simulink model "Square_HFI"  (R2022b)
settings: Solver=FixedStepAuto  StartTime=0.0  StopTime=10  FixedStep=1e-5  RelTol=1e-3
undefined symbols (not defined in the file): curr_d_ki, curr_d_kp, curr_q_ki, curr_q_kp, CurrKi, CurrKpd, CurrKpq, DiscIntNeverNeededParam, Ld, Lq, PLL_Kd, PLL_Ki, Pn, sigbuilder_block, spd_ki, spd_kp
libraries: dsparch4 x4, slpidlib x3, mcbplantlib x1, autolibpmsminterior x1, autolibpmsmexterior x1
settings Model: DataDictionary=Square_HFI.sldd  Creator=SSC  LastModifiedBy=SSC
settings GRTTargetCC: RTWCAPISignals=on  RTWCAPIParams=on

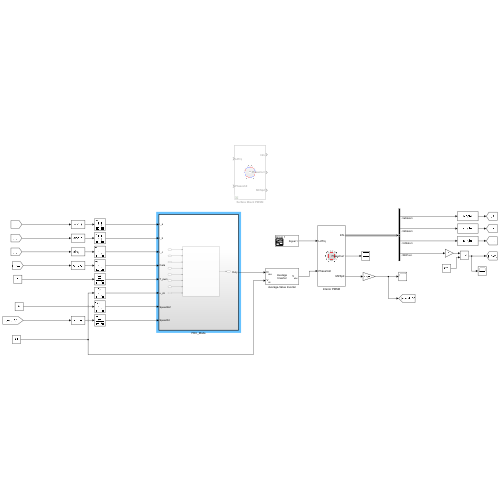
[thumbnail: Simulink's stored preview of the top-level diagram]
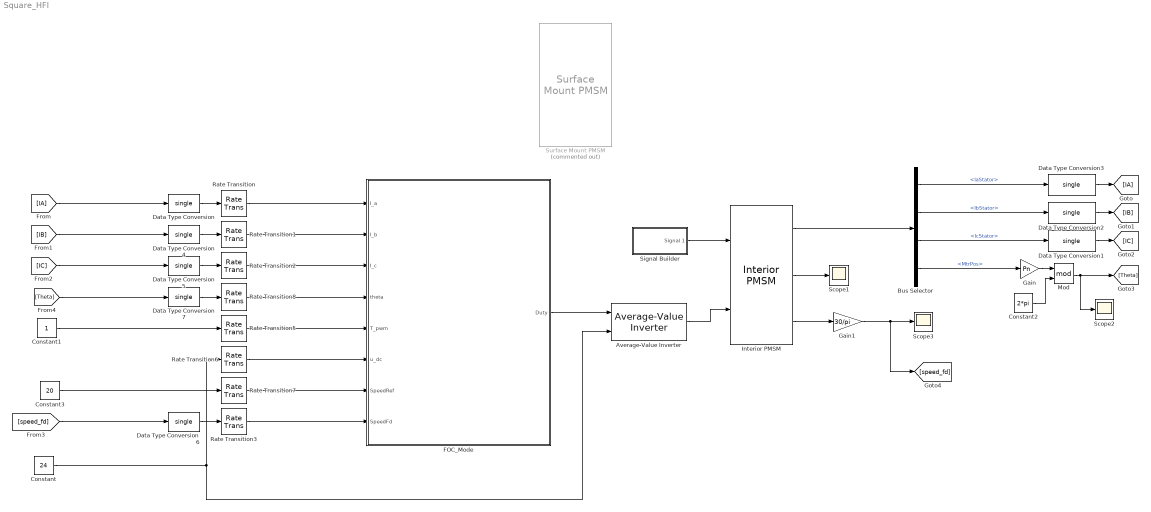
== system Square_HFI ==
  Average-Value Inverter : mcbplantlib/Average-Value Inverter
      settings: LibrarySourceBlock=mcblib/Electrical Systems/Inverters/Average-Value Inverter
  Bus Selector : BusSelector  OutputSignals=IaStator,IbStator,IcStator,MtrPos
  Constant : Constant  Value=24  OutDataTypeStr=single
  Constant1 : Constant  OutDataTypeStr=single
  Constant2 : Constant  Value=2*pi  OutDataTypeStr=single
  Constant3 : Constant  Value=20  OutDataTypeStr=single
  Data Type Conversion{,1..7} (8 alike) : DataTypeConversion  OutDataTypeStr=single  SaturateOnIntegerOverflow=off  RndMeth=Floor
  FOC_Mode : Subsystem  TreatAsAtomicUnit=on
  Gain : Gain  Gain=Pn  OutDataTypeStr=single
  Gain1 : Gain  Gain=30/pi  OutDataTypeStr=single
  Interior PMSM : autolibpmsminterior/Interior PMSM  port_config=Torque  sim_type=Discrete  Ts=1e-4  P=Pn  Rs=Rs  Ldq=[Ld Lq]  KConstText=Permanent flux linkage constant (lambda_pm):  lambda_pm=flux  Ke=159.9771  mechanical=[75e-6,8e-5,0]  idq0=[0 0]  theta_init=0  omega_init=0  KConst=flux  lambda_pm_calc=flux  Kt=0.07  RefBlkName='autolibpmsminterior/Interior PMSM'  aMode=5
      settings: LibrarySourceBlock=mcblib/Electrical Systems/Motors/Interior PMSM
  Mod : Math  Operator=mod
  Rate Transition{,1..3,5..8} (8 alike) : RateTransition
  Scope1 : Scope
  Scope2 : Scope
  Scope3 : Scope
  Signal Builder : Subsystem  Tag=STV Subsys  LoadFcn=sigbuilder_block('load');  StartFcn=sigbuilder_block('start');  StopFcn=sigbuilder_block('stop');  ClipboardFcn=sigbuilder_block('clipboard');  mask(Sigbuilder block){tuvar=[0:10]}
      mask help: Simulink:masks:SigbuilderBlock_MD
      mask init:
      | if ~strcmp(get_param(bdroot(gcbh),'SimulationStatus'),'stopped') tuvar = sigbuilder_block('maskInit'); end
      settings: CopyFcn=sigbuilder_block('copy');  DeleteFcn=sigbuilder_block('delete');  ModelCloseFcn=sigbuilder_block('modelClose');  PreSaveFcn=sigbuilder_block('preSave');  PauseFcn=sigbuilder_block('pause');  ContinueFcn=sigbuilder_block('continue');  NameChangeFcn=sigbuilder_block('namechange');  OpenFcn=sigbuilder_block('open',[367.2 103.2 550.8 400.2 ]);  CloseFcn=sigbuilder_block('close');
      mask Display: plot(0, 0, 100, 100,[2, 2, 32, 32, 2], [68, 8, 8, 68, 68],[32, 2], [38, 38], [32, 19, 2],[53, 60, 44], [32, 17, 17, 2],[16, 16, 31, 31]);txt = getActiveGroup(gcbh);text(2, 100, txt,'verticalAlignment', 'top');
  Surface Mount PMSM : autolibpmsmexterior/Surface Mount PMSM  Commented=on  port_config=Torque  sim_type=Discrete  Ts=1e-4  P=Pn  Rs=Rs  Ldq_=Ld  KConstText=Permanent flux linkage constant (lambda_pm):  lambda_pm=flux  Ke=223  Kt=1.323  mechanical=[75e-6,8e-5,0]  idq0=[0 0]  theta_init=0  omega_init=0  KConst=flux  lambda_pm_calc=flux  RefBlkName='autolibpmsmexterior/Surface Mount PMSM'  aMode=5  Ldq="[0.0017      0.0017]"
  wires:
  Rate Transition/1 -> FOC_Mode/1(I_a)
  Average-Value Inverter/1 -> Interior PMSM/2
  Rate Transition7/1 -> FOC_Mode/7(SpeedRef)
  Data Type Conversion6/1 -> Rate Transition3/1
  [IC] -> Data Type Conversion5/1
  Data Type Conversion5/1 -> Rate Transition2/1
  Data Type Conversion2/1 -> [IB]
  Rate Transition1/1 -> FOC_Mode/2(I_b)
  Interior PMSM/2 -> Scope1/1
  Bus Selector/3 -> Data Type Conversion1/1  "<IcStator>"
  Rate Transition6/1 -> FOC_Mode/6(u_dc)
  Constant1/1 -> Rate Transition5/1
  Bus Selector/4 -> Gain/1  "<MtrPos>"
  FOC_Mode/1(Duty) -> Average-Value Inverter/1
  [IA] -> Data Type Conversion/1
  Gain1/1 -> Scope3/1, [speed_fd]
  Rate Transition8/1 -> FOC_Mode/4(theta)
  Bus Selector/2 -> Data Type Conversion2/1  "<IbStator>"
  Data Type Conversion/1 -> Rate Transition/1
  Interior PMSM/1 -> Bus Selector/1
  Data Type Conversion3/1 -> [IA]
  Interior PMSM/3 -> Gain1/1
  Constant3/1 -> Rate Transition7/1
  Gain/1 -> Mod/1
  [Theta] -> Data Type Conversion7/1
  Rate Transition2/1 -> FOC_Mode/3(I_c)
  Data Type Conversion4/1 -> Rate Transition1/1
  Bus Selector/1 -> Data Type Conversion3/1  "<IaStator>"
  [speed_fd] -> Data Type Conversion6/1
  Data Type Conversion7/1 -> Rate Transition8/1
  Mod/1 -> Scope2/1, [Theta]
  Rate Transition3/1 -> FOC_Mode/8(SpeedFd)
  Constant/1 -> Average-Value Inverter/2, Rate Transition6/1
  Constant2/1 -> Mod/2
  Data Type Conversion1/1 -> [IC]
  Rate Transition5/1 -> FOC_Mode/5(T_pwm)
  [IB] -> Data Type Conversion4/1
  Signal Builder/1(Signal 1) -> Interior PMSM/1

== system Square_HFI/FOC_Mode ==
  I_a : Inport
  I_b : Inport  Port=2
  I_c : Inport  Port=3
  theta : Inport  Port=4
  T_pwm : Inport  Port=5
  u_dc : Inport  Port=6
  SpeedRef : Inport  Port=7
  SpeedFd : Inport  Port=8
  HFI_Mode : Subsystem  TreatAsAtomicUnit=on
  Duty : Outport
  wires:
  T_pwm/1 -> HFI_Mode/5(T_pwm)
  u_dc/1 -> HFI_Mode/6(u_dc)
  HFI_Mode/1(Duty) -> Duty/1
  I_a/1 -> HFI_Mode/1(I_a)
  I_b/1 -> HFI_Mode/2(I_b)
  I_c/1 -> HFI_Mode/3(I_c)
  theta/1 -> HFI_Mode/4(theta)
  SpeedRef/1 -> HFI_Mode/7(SpeedRef)
  SpeedFd/1 -> HFI_Mode/8(SpeedFd)

== system Square_HFI/Signal Builder ==
  Demux : Demux  Tag=STV Demux  Outputs=1
      settings: DisplayOption=none
  FromWs : FromWorkspace  Tag=STV FromWs  VariableName=tuvar
      SigBuilderData=|
      | common.afterFinalStr = 'Extrapolate'
      | common.sampleTime = 0
      | dataSet.timeRange = [0 10]
      | dataSet.name = 'Group 1'
      | sbobj.Groups.Name = 'Group 1'
      | sbobj.Groups.Signals.Name = 'Signal 1'
      | sbobj.Groups.Signals.XData = [0 4 4 6 10]
      | sbobj.Groups.Signals.YData = [0 0 0.0003 0.0003 0.0003]
  Signal 1 : Outport  Tag=STV Outport
  wires:
  Demux/1 -> Signal 1/1
  FromWs/1 -> Demux/1

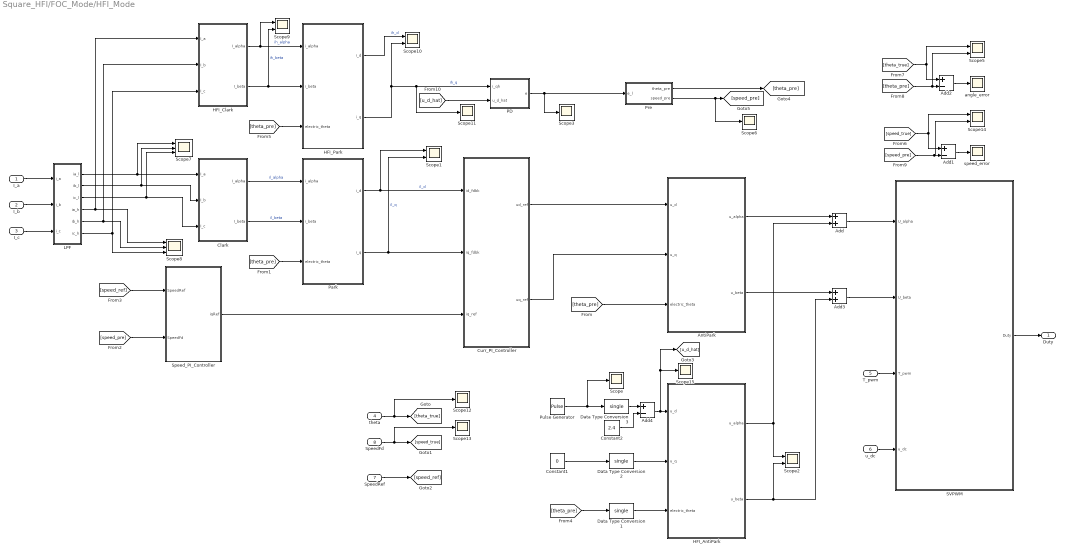
== system Square_HFI/FOC_Mode/HFI_Mode ==
  I_a : Inport
  I_b : Inport  Port=2
  I_c : Inport  Port=3
  theta : Inport  Port=4
  T_pwm : Inport  Port=5
  u_dc : Inport  Port=6
  SpeedRef : Inport  Port=7
  SpeedFd : Inport  Port=8
  Add : Sum  OutDataTypeStr=single
  Add1 : Sum  Inputs=+-  OutDataTypeStr=single
  Add2 : Sum  Inputs=+-  OutDataTypeStr=single
  Add3 : Sum  OutDataTypeStr=single
  Add4 : Sum  Inputs=+-  OutDataTypeStr=single
  AntiPark : Subsystem
  Clark : Subsystem
  Constant1 : Constant  Value=0  OutDataTypeStr=single
  Constant2 : Constant  Value=2.4  OutDataTypeStr=single
  Curr_PI_Controller : Subsystem
  Data Type Conversion1 : DataTypeConversion  OutDataTypeStr=single  SaturateOnIntegerOverflow=off  RndMeth=Floor
  Data Type Conversion2 : DataTypeConversion  OutDataTypeStr=single  SaturateOnIntegerOverflow=off  RndMeth=Floor
  Data Type Conversion3 : DataTypeConversion  OutDataTypeStr=single  SaturateOnIntegerOverflow=off  RndMeth=Floor
  HFI_AntiPark : Subsystem
  HFI_Clark : Subsystem
  HFI_Park : Subsystem
  LPF : Subsystem
  PD : Subsystem
  Park : Subsystem
  Pre : Subsystem
  Pulse Generator : DiscretePulseGenerator  PulseType=Time based  Amplitude=4.8  Period=0.001  PulseWidth=50
  SVPWM : Subsystem
  Scope{,3,6,11..13,15} (7 alike) : Scope
  Scope{1..2,5,9..10,14} (6 alike) : Scope  NumInputPorts=2
  Scope7 : Scope  NumInputPorts=3
  Scope8 : Scope  NumInputPorts=3
  Speed_PI_Controller : Subsystem
  angle_error : Scope
  speed_error : Scope
  Duty : Outport
  wires:
  Curr_PI_Controller/2(uq_ref) -> AntiPark/2(u_q)
  SVPWM/1(Duty) -> Duty/1
  u_dc/1 -> SVPWM/4(u_dc)
  T_pwm/1 -> SVPWM/3(T_pwm)
  Curr_PI_Controller/1(ud_ref) -> AntiPark/1(u_d)
  PD/1(e) -> Pre/1(e_l), Scope3/1
  Pulse Generator/1 -> Scope/1, Data Type Conversion3/1
  Add/1 -> SVPWM/1(U_alpha)
  Add3/1 -> SVPWM/2(U_beta)
  Constant1/1 -> Data Type Conversion2/1
  I_b/1 -> LPF/2(i_b)
  I_a/1 -> LPF/1(i_a)
  I_c/1 -> LPF/3(i_c)
  AntiPark/1(u_alpha) -> Add/1
  AntiPark/2(u_beta) -> Add3/1
  theta/1 -> Scope12/1, [theta_true]
  SpeedFd/1 -> Scope13/1, [speed_true]
  Park/1(i_d) -> Scope1/1, Curr_PI_Controller/1(id_fdbk)  "il_d"
  Park/2(i_q) -> Scope1/2, Curr_PI_Controller/2(iq_fdbk)  "il_q"
  Speed_PI_Controller/1(iqRef) -> Curr_PI_Controller/3(iq_ref)
  [theta_pre] -> AntiPark/3(electric_theta)
  Clark/1(I_alpha) -> Park/1(i_alpha)  "il_alpha"
  Clark/2(I_beta) -> Park/2(i_beta)  "il_beta"
  [theta_pre] -> Park/3(electric_theta)
  LPF/1(ia_l) -> Scope7/1, Clark/1(I_a)
  LPF/3(ic_l) -> Scope7/3, Clark/3(I_c)
  LPF/2(ib_l) -> Scope7/2, Clark/2(I_b)
  [speed_pre] -> Speed_PI_Controller/2(SpeedFd)
  SpeedRef/1 -> [speed_ref]
  [speed_ref] -> Speed_PI_Controller/1(SpeedRef)
  [theta_pre] -> Data Type Conversion1/1
  HFI_AntiPark/1(u_alpha) -> Add/2, Scope2/1
  HFI_AntiPark/2(u_beta) -> Add3/2, Scope2/2
  LPF/4(ia_h) -> HFI_Clark/1(I_a), Scope8/1
  LPF/5(ib_h) -> HFI_Clark/2(I_b), Scope8/2
  LPF/6(ic_h) -> Scope8/3, HFI_Clark/3(I_c)
  HFI_Clark/1(I_alpha) -> HFI_Park/1(i_alpha), Scope9/1  "ih_alpha"
  HFI_Clark/2(I_beta) -> HFI_Park/2(i_beta), Scope9/2  "ih_beta"
  [theta_pre] -> HFI_Park/3(electric_theta)
  HFI_Park/1(i_d) -> Scope10/1  "ih_d"
  HFI_Park/2(i_q) -> Scope10/2, Scope11/1, PD/1(i_qh)  "ih_q"
  Pre/2(speed_pre) -> Scope6/1, [speed_pre]
  Pre/1(theta_pre) -> [theta_pre]
  [theta_pre] -> Scope5/2, Add2/2
  [theta_true] -> Add2/1, Scope5/1
  Add2/1 -> angle_error/1
  Data Type Conversion1/1 -> HFI_AntiPark/3(electric_theta)
  Data Type Conversion2/1 -> HFI_AntiPark/2(u_q)
  [speed_true] -> Scope14/1, Add1/1
  [speed_pre] -> Scope14/2, Add1/2
  Add1/1 -> speed_error/1
  Data Type Conversion3/1 -> Add4/1
  Add4/1 -> [u_d_hat], Scope15/1, HFI_AntiPark/1(u_d)
  Constant2/1 -> Add4/2
  [u_d_hat] -> PD/2(u_d_hat)

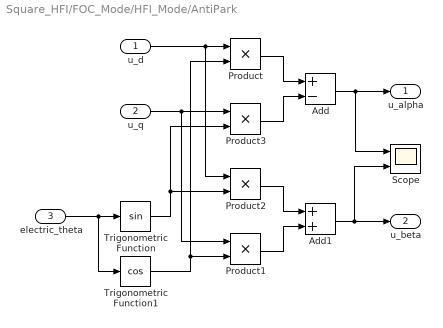
== system Square_HFI/FOC_Mode/HFI_Mode/AntiPark ==
  u_d : Inport
  u_q : Inport  Port=2
  electric_theta : Inport  Port=3
  Add : Sum  Inputs=+-
  Add1 : Sum
  Product{,1..3} (4 alike) : Product
  Scope : Scope  NumInputPorts=2
  Trigonometric Function : Trigonometry
  Trigonometric Function1 : Trigonometry  Operator=cos
  u_alpha : Outport
  u_beta : Outport  Port=2
  wires:
  electric_theta/1 -> Trigonometric Function1/1, Trigonometric Function/1
  u_d/1 -> Product2/1, Product/1
  Trigonometric Function1/1 -> Product/2, Product1/2
  u_q/1 -> Product1/1, Product3/1
  Trigonometric Function/1 -> Product2/2, Product3/2
  Product/1 -> Add/1
  Product3/1 -> Add/2
  Add/1 -> Scope/1, u_alpha/1
  Product2/1 -> Add1/1
  Product1/1 -> Add1/2
  Add1/1 -> Scope/2, u_beta/1

== system Square_HFI/FOC_Mode/HFI_Mode/Clark ==
  I_a : Inport
  I_b : Inport  Port=2
  I_c : Inport  Port=3
  Add : Sum
  Add1 : Sum  Inputs=+-
  Add2 : Sum  Inputs=+-
  Gain : Gain  Gain=2/3
  Gain1 : Gain  Gain=1/3
  Gain2 : Gain  Gain=sqrt(3)/3
  I_alpha : Outport
  I_beta : Outport  Port=2
  wires:
  I_a/1 -> Gain/1
  I_b/1 -> Add1/1, Add/1
  I_c/1 -> Add/2, Add1/2
  Add/1 -> Gain1/1
  Add1/1 -> Gain2/1
  Gain/1 -> Add2/1
  Gain1/1 -> Add2/2
  Add2/1 -> I_alpha/1
  Gain2/1 -> I_beta/1

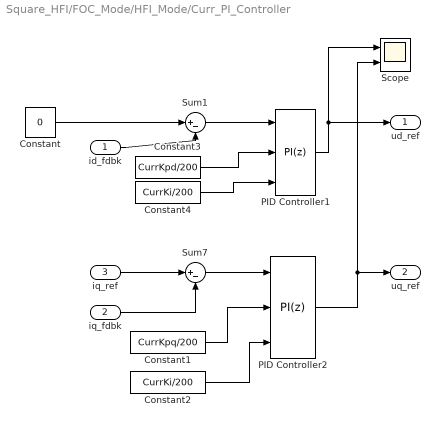
== system Square_HFI/FOC_Mode/HFI_Mode/Curr_PI_Controller ==
  id_fdbk : Inport  OutDataTypeStr=single
  iq_fdbk : Inport  Port=2  OutDataTypeStr=single
  iq_ref : Inport  Port=3  OutDataTypeStr=single
  Constant : Constant  Value=0  OutDataTypeStr=single
  Constant1 : Constant  Value=CurrKpq/200  OutDataTypeStr=single
  Constant2 : Constant  Value=CurrKi/200  OutDataTypeStr=single
  Constant3 : Constant  Value=CurrKpd/200  OutDataTypeStr=single
  Constant4 : Constant  Value=CurrKi/200  OutDataTypeStr=single
  PID Controller1 : slpidlib/PID Controller  Controller=PI  Form=Parallel  TimeDomain=Discrete-time  UseExternalTs=off  SampleTime=-1  IntegratorMethod=Forward Euler  FilterMethod=Forward Euler  ControllerParametersSource=external  P=curr_d_kp  I=curr_d_ki  UseKiTs=off  D=0  N=100  UseFilter=on  TunerSelectOption=Transfer Function Based (PID Tuner App)  InitialConditionSource=internal  InitialConditionForIntegrator=0  InitialConditionForFilter=0  DifferentiatorICPrevScaledInput=0  ExternalReset=none  TrackingMode=off  Kt=1  LimitOutput=on  SatLimitsSource=internal  UpperSaturationLimit=24*0.9/sqrt(3)  LowerSaturationLimit=-24*0.9/sqrt(3)  LinearizeAsGain=on  AntiWindupMode=clamping  Kb=1  LimitIntegrator=off  UpperIntegratorSaturationLimit=inf  LowerIntegratorSaturationLimit=-inf  PGainOutDataTypeStr=single  PProdOutDataTypeStr=single  POutMin=[]  POutMax=[]  IGainOutDataTypeStr=int16  IProdOutDataTypeStr=int16  IOutMin=[]  IOutMax=[]  DOutMin=[]  DOutMax=[]  NOutMin=[]  NOutMax=[]  SumOutDataTypeStr=single  SumOutMin=[]  SumOutMax=[]  SaturationOutDataTypeStr=single  SaturationOutMin=[]  SaturationOutMax=[]  PParamMin=[]  PParamMax=[]  IParamMin=[]  IParamMax=[]  DParamMin=[]  DParamMax=[]  NParamMin=[]  NParamMax=[]  KbParamMin=[]  KbParamMax=[]  KtParamMin=[]  KtParamMax=[]  KbOutMin=[]  KbOutMax=[]  KtOutMin=[]  KtOutMax=[]  IntegratorOutMin=[]  IntegratorOutMax=[]  FilterOutMin=[]  FilterOutMax=[]  SumI1OutMin=[]  SumI1OutMax=[]  SumI2OutMin=[]  SumI2OutMax=[]  SumI3OutMin=[]  SumI3OutMax=[]  SumI4OutMin=[]  SumI4OutMax=[]  SumDOutMin=[]  SumDOutMax=[]  DifferentiatorOutMin=[]  DifferentiatorOutMax=[]  FilterDiffOutCoefMin=[]  FilterDiffOutCoefMax=[]  ReciprocalOutMin=[]  ReciprocalOutMax=[]  SumDenOutMin=[]  SumDenOutMax=[]  SumNumOutMin=[]  SumNumOutMax=[]  DivideOutMin=[]  DivideOutMax=[]  UdiffTsProdOutMin=[]  UdiffTsProdOutMax=[]  NTsProdOutMin=[]  NTsProdOutMax=[]  UintegralTsProdOutMin=[]  UintegralTsProdOutMax=[]  UngainTsProdOutMin=[]  UngainTsProdOutMax=[]  ClampingZeroOutDataTypeStr=Inherit: Inherit via back propagation  ClampingZeroOutMin=[]  ClampingZeroOutMax=[]  FilterDenConstantOutDataTypeStr=Inherit: Inherit via back propagation  FilterDenConstantOutMin=[]  FilterDenConstantOutMax=[]  PCopyOutDataTypeStr=Inherit: Inherit via back propagation  PCopyOutMin=[]  PCopyOutMax=[]  NCopyOutDataTypeStr=Inherit: Inherit via back propagation  NCopyOutMin=[]  NCopyOutMax=[]  IntegratorContinuousStateAttributes=''  IntegratorStateMustResolveToSignalObject=off  IntegratorRTWStateStorageClass=Auto  FilterContinuousStateAttributes=''  FilterStateMustResolveToSignalObject=off  FilterRTWStateStorageClass=Auto  ParallelPVariant=ExternalParameters  IdealPVariant=Disabled  IVariant=ExternalParameters  DVariant=Disabled  IntegratorVariant=Discrete  SatVariant=Enabled  AWVariant=DiscClampingParallel  PCopyVariant=Disabled  TRVariant=Disabled  FdbkBlocksVariant=Forward  IdealPFdbkVariant=Disabled  SatFdbkVariant=Disabled  DerivativeFilterVariant=Disabled  NVariant=Disabled  NCopyVariant=Disabled_SignalSpec  FilterICVariant=Disabled  IntegratorICVariant=InternalICs  ExternalResetVariant=Disabled  TRSumVariant=Passthrough  SumFdbkVariant=Disabled  SumVariant=Sum_PI  TsampFilterVariant=InternalTs  TsampNgainVariant=Passthrough  TsampIntegralVariant=Passthrough  ExternalSaturationOutDataTypeStr=Inherit: Same as second input
  PID Controller2 : slpidlib/PID Controller  Controller=PI  Form=Parallel  TimeDomain=Discrete-time  UseExternalTs=off  SampleTime=-1  IntegratorMethod=Forward Euler  FilterMethod=Forward Euler  ControllerParametersSource=external  P=curr_q_kp  I=curr_q_ki  UseKiTs=off  D=0  N=100  UseFilter=on  TunerSelectOption=Transfer Function Based (PID Tuner App)  InitialConditionSource=internal  InitialConditionForIntegrator=0  InitialConditionForFilter=0  DifferentiatorICPrevScaledInput=0  ExternalReset=none  TrackingMode=off  Kt=1  LimitOutput=on  SatLimitsSource=internal  UpperSaturationLimit=24*0.9/sqrt(3)  LowerSaturationLimit=-24*0.9/sqrt(3)  LinearizeAsGain=on  AntiWindupMode=clamping  Kb=1  LimitIntegrator=off  UpperIntegratorSaturationLimit=inf  LowerIntegratorSaturationLimit=-inf  PGainOutDataTypeStr=single  PProdOutDataTypeStr=single  POutMin=[]  POutMax=[]  IGainOutDataTypeStr=single  IProdOutDataTypeStr=single  IOutMin=[]  IOutMax=[]  DOutMin=[]  DOutMax=[]  NOutMin=[]  NOutMax=[]  SumOutDataTypeStr=single  SumOutMin=[]  SumOutMax=[]  SaturationOutDataTypeStr=single  SaturationOutMin=[]  SaturationOutMax=[]  PParamMin=[]  PParamMax=[]  IParamMin=[]  IParamMax=[]  DParamMin=[]  DParamMax=[]  NParamMin=[]  NParamMax=[]  KbParamMin=[]  KbParamMax=[]  KtParamMin=[]  KtParamMax=[]  KbOutMin=[]  KbOutMax=[]  KtOutMin=[]  KtOutMax=[]  IntegratorOutMin=[]  IntegratorOutMax=[]  FilterOutMin=[]  FilterOutMax=[]  SumI1OutMin=[]  SumI1OutMax=[]  SumI2OutMin=[]  SumI2OutMax=[]  SumI3OutMin=[]  SumI3OutMax=[]  SumI4OutMin=[]  SumI4OutMax=[]  SumDOutMin=[]  SumDOutMax=[]  DifferentiatorOutMin=[]  DifferentiatorOutMax=[]  FilterDiffOutCoefMin=[]  FilterDiffOutCoefMax=[]  ReciprocalOutMin=[]  ReciprocalOutMax=[]  SumDenOutMin=[]  SumDenOutMax=[]  SumNumOutMin=[]  SumNumOutMax=[]  DivideOutMin=[]  DivideOutMax=[]  UdiffTsProdOutMin=[]  UdiffTsProdOutMax=[]  NTsProdOutMin=[]  NTsProdOutMax=[]  UintegralTsProdOutMin=[]  UintegralTsProdOutMax=[]  UngainTsProdOutMin=[]  UngainTsProdOutMax=[]  ClampingZeroOutDataTypeStr=Inherit: Inherit via back propagation  ClampingZeroOutMin=[]  ClampingZeroOutMax=[]  FilterDenConstantOutDataTypeStr=Inherit: Inherit via back propagation  FilterDenConstantOutMin=[]  FilterDenConstantOutMax=[]  PCopyOutDataTypeStr=Inherit: Inherit via back propagation  PCopyOutMin=[]  PCopyOutMax=[]  NCopyOutDataTypeStr=Inherit: Inherit via back propagation  NCopyOutMin=[]  NCopyOutMax=[]  IntegratorContinuousStateAttributes=''  IntegratorStateMustResolveToSignalObject=off  IntegratorRTWStateStorageClass=Auto  FilterContinuousStateAttributes=''  FilterStateMustResolveToSignalObject=off  FilterRTWStateStorageClass=Auto  ParallelPVariant=ExternalParameters  IdealPVariant=Disabled  IVariant=ExternalParameters  DVariant=Disabled  IntegratorVariant=Discrete  SatVariant=Enabled  AWVariant=DiscClampingParallel  PCopyVariant=Disabled  TRVariant=Disabled  FdbkBlocksVariant=Forward  IdealPFdbkVariant=Disabled  SatFdbkVariant=Disabled  DerivativeFilterVariant=Disabled  NVariant=Disabled  NCopyVariant=Disabled_SignalSpec  FilterICVariant=Disabled  IntegratorICVariant=InternalICs  ExternalResetVariant=Disabled  TRSumVariant=Passthrough  SumFdbkVariant=Disabled  SumVariant=Sum_PI  TsampFilterVariant=InternalTs  TsampNgainVariant=Passthrough  TsampIntegralVariant=Passthrough  ExternalSaturationOutDataTypeStr=Inherit: Same as second input
  Scope : Scope  NumInputPorts=2
  Sum1 : Sum  Inputs=|+-  AccumDataTypeStr=single  OutDataTypeStr=single
  Sum7 : Sum  Inputs=|+-  AccumDataTypeStr=single  OutDataTypeStr=single
  ud_ref : Outport  OutDataTypeStr=single
  uq_ref : Outport  Port=2  OutDataTypeStr=single
  wires:
  id_fdbk/1 -> Sum1/2
  Constant/1 -> Sum1/1
  iq_fdbk/1 -> Sum7/2
  Sum1/1 -> PID Controller1/1
  PID Controller1/1 -> Scope/1, ud_ref/1
  PID Controller2/1 -> Scope/2, uq_ref/1
  iq_ref/1 -> Sum7/1
  Constant3/1 -> PID Controller1/2
  Constant4/1 -> PID Controller1/3
  Constant1/1 -> PID Controller2/2
  Constant2/1 -> PID Controller2/3
  Sum7/1 -> PID Controller2/1

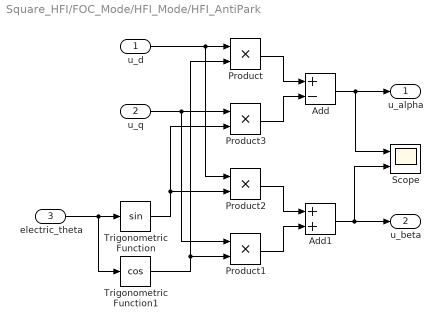
== system Square_HFI/FOC_Mode/HFI_Mode/HFI_AntiPark ==
  u_d : Inport
  u_q : Inport  Port=2
  electric_theta : Inport  Port=3
  Add : Sum  Inputs=+-
  Add1 : Sum
  Product{,1..3} (4 alike) : Product
  Scope : Scope  NumInputPorts=2
  Trigonometric Function : Trigonometry
  Trigonometric Function1 : Trigonometry  Operator=cos
  u_alpha : Outport
  u_beta : Outport  Port=2
  wires:
  electric_theta/1 -> Trigonometric Function1/1, Trigonometric Function/1
  u_d/1 -> Product2/1, Product/1
  Trigonometric Function1/1 -> Product/2, Product1/2
  u_q/1 -> Product1/1, Product3/1
  Trigonometric Function/1 -> Product2/2, Product3/2
  Product/1 -> Add/1
  Product3/1 -> Add/2
  Add/1 -> Scope/1, u_alpha/1
  Product2/1 -> Add1/1
  Product1/1 -> Add1/2
  Add1/1 -> Scope/2, u_beta/1

== system Square_HFI/FOC_Mode/HFI_Mode/HFI_Clark ==
  I_a : Inport
  I_b : Inport  Port=2
  I_c : Inport  Port=3
  Add : Sum
  Add1 : Sum  Inputs=+-
  Add2 : Sum  Inputs=+-
  Gain : Gain  Gain=2/3
  Gain1 : Gain  Gain=1/3
  Gain2 : Gain  Gain=sqrt(3)/3
  I_alpha : Outport
  I_beta : Outport  Port=2
  wires:
  I_a/1 -> Gain/1
  I_b/1 -> Add1/1, Add/1
  I_c/1 -> Add/2, Add1/2
  Add/1 -> Gain1/1
  Add1/1 -> Gain2/1
  Gain/1 -> Add2/1
  Gain1/1 -> Add2/2
  Add2/1 -> I_alpha/1
  Gain2/1 -> I_beta/1

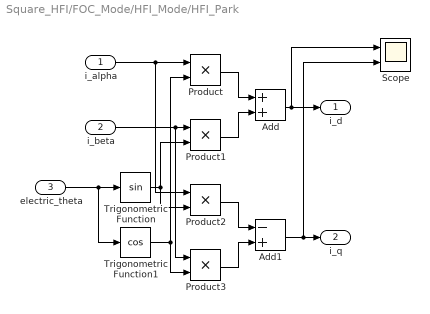
== system Square_HFI/FOC_Mode/HFI_Mode/HFI_Park ==
  i_alpha : Inport
  i_beta : Inport  Port=2
  electric_theta : Inport  Port=3
  Add : Sum
  Add1 : Sum  Inputs=-+
  Product{,1..3} (4 alike) : Product
  Scope : Scope  NumInputPorts=2
  Trigonometric Function : Trigonometry
  Trigonometric Function1 : Trigonometry  Operator=cos
  i_d : Outport
  i_q : Outport  Port=2
  wires:
  electric_theta/1 -> Trigonometric Function1/1, Trigonometric Function/1
  i_alpha/1 -> Product2/1, Product/1
  Trigonometric Function1/1 -> Product3/2, Product/2
  i_beta/1 -> Product3/1, Product1/1
  Trigonometric Function/1 -> Product2/2, Product1/2
  Product/1 -> Add/1
  Product1/1 -> Add/2
  Product2/1 -> Add1/1
  Product3/1 -> Add1/2
  Add/1 -> Scope/1, i_d/1
  Add1/1 -> Scope/2, i_q/1

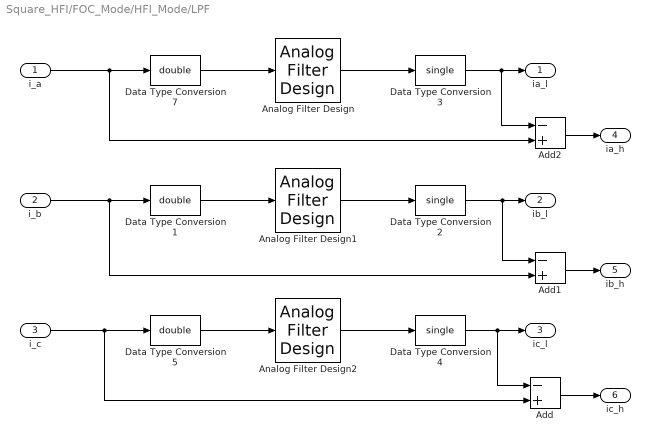
== system Square_HFI/FOC_Mode/HFI_Mode/LPF ==
  i_a : Inport
  i_b : Inport  Port=2
  i_c : Inport  Port=3
  Add : Sum  Inputs=-+
  Add1 : Sum  Inputs=-+
  Add2 : Sum  Inputs=-+
  Analog Filter Design : dsparch4/Analog Filter Design  method=Butterworth  filttype=Lowpass  N=3  Wlo=100*pi  Whi=80  Rp=2  Rs=40
  Analog Filter Design1 : dsparch4/Analog Filter Design  method=Butterworth  filttype=Lowpass  N=3  Wlo=100*pi  Whi=80  Rp=2  Rs=40
  Analog Filter Design2 : dsparch4/Analog Filter Design  method=Butterworth  filttype=Lowpass  N=3  Wlo=100*pi  Whi=80  Rp=2  Rs=40
  Data Type Conversion1 : DataTypeConversion  OutDataTypeStr=double  SaturateOnIntegerOverflow=off  RndMeth=Floor
  Data Type Conversion2 : DataTypeConversion  OutDataTypeStr=single  SaturateOnIntegerOverflow=off  RndMeth=Floor
  Data Type Conversion3 : DataTypeConversion  OutDataTypeStr=single  SaturateOnIntegerOverflow=off  RndMeth=Floor
  Data Type Conversion4 : DataTypeConversion  OutDataTypeStr=single  SaturateOnIntegerOverflow=off  RndMeth=Floor
  Data Type Conversion5 : DataTypeConversion  OutDataTypeStr=double  SaturateOnIntegerOverflow=off  RndMeth=Floor
  Data Type Conversion7 : DataTypeConversion  OutDataTypeStr=double  SaturateOnIntegerOverflow=off  RndMeth=Floor
  ia_l : Outport
  ib_l : Outport  Port=2
  ic_l : Outport  Port=3
  ia_h : Outport  Port=4
  ib_h : Outport  Port=5
  ic_h : Outport  Port=6
  wires:
  Analog Filter Design1/1 -> Data Type Conversion2/1
  Analog Filter Design/1 -> Data Type Conversion3/1
  Data Type Conversion7/1 -> Analog Filter Design/1
  Data Type Conversion1/1 -> Analog Filter Design1/1
  Data Type Conversion5/1 -> Analog Filter Design2/1
  Analog Filter Design2/1 -> Data Type Conversion4/1
  i_c/1 -> Add/2, Data Type Conversion5/1
  Data Type Conversion4/1 -> Add/1, ic_l/1
  Add/1 -> ic_h/1
  Data Type Conversion2/1 -> Add1/1, ib_l/1
  i_b/1 -> Add1/2, Data Type Conversion1/1
  Add1/1 -> ib_h/1
  Data Type Conversion3/1 -> Add2/1, ia_l/1
  i_a/1 -> Add2/2, Data Type Conversion7/1
  Add2/1 -> ia_h/1

== system Square_HFI/FOC_Mode/HFI_Mode/PD ==
  i_qh : Inport
  u_d_hat : Inport  Port=2
  Add : Sum  Inputs=-+
  Delay : Delay  DelayLength=10  InitialCondition=0
  Product : Product
  Scope : Scope
  Scope1 : Scope  NumInputPorts=2
  Sign : Signum
  Zero-Order Hold : ZeroOrderHold  SampleTime=-1
  e : Outport
  wires:
  Product/1 -> e/1
  Delay/1 -> Scope1/1, Add/1
  Sign/1 -> Product/2, Scope/1
  u_d_hat/1 -> Sign/1
  i_qh/1 -> Scope1/2, Add/2, Delay/1
  Add/1 -> Zero-Order Hold/1
  Zero-Order Hold/1 -> Product/1

== system Square_HFI/FOC_Mode/HFI_Mode/Park ==
  i_alpha : Inport
  i_beta : Inport  Port=2
  electric_theta : Inport  Port=3
  Add : Sum
  Add1 : Sum  Inputs=-+
  Product{,1..3} (4 alike) : Product
  Scope : Scope  NumInputPorts=2
  Trigonometric Function : Trigonometry
  Trigonometric Function1 : Trigonometry  Operator=cos
  i_d : Outport
  i_q : Outport  Port=2
  wires:
  electric_theta/1 -> Trigonometric Function1/1, Trigonometric Function/1
  i_alpha/1 -> Product2/1, Product/1
  Trigonometric Function1/1 -> Product3/2, Product/2
  i_beta/1 -> Product3/1, Product1/1
  Trigonometric Function/1 -> Product2/2, Product1/2
  Product/1 -> Add/1
  Product1/1 -> Add/2
  Product2/1 -> Add1/1
  Product3/1 -> Add1/2
  Add/1 -> Scope/1, i_d/1
  Add1/1 -> Scope/2, i_q/1

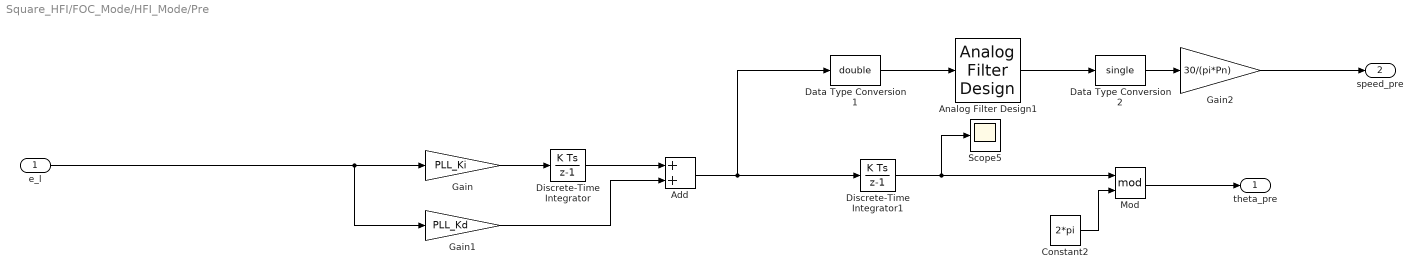
== system Square_HFI/FOC_Mode/HFI_Mode/Pre ==
  e_l : Inport
  Add : Sum
  Analog Filter Design1 : dsparch4/Analog Filter Design  method=Butterworth  filttype=Lowpass  N=4  Wlo=100*pi  Whi=80  Rp=2  Rs=40
  Constant2 : Constant  Value=2*pi  OutDataTypeStr=single
  Data Type Conversion1 : DataTypeConversion  OutDataTypeStr=double  SaturateOnIntegerOverflow=off  RndMeth=Floor
  Data Type Conversion2 : DataTypeConversion  OutDataTypeStr=single  SaturateOnIntegerOverflow=off  RndMeth=Floor
  Discrete-Time Integrator : DiscreteIntegrator  SampleTime=-1  OutDataTypeStr=single  ICPrevOutput=DiscIntNeverNeededParam  ICPrevScaledInput=DiscIntNeverNeededParam
  Discrete-Time Integrator1 : DiscreteIntegrator  SampleTime=-1  OutDataTypeStr=single  ICPrevOutput=DiscIntNeverNeededParam  ICPrevScaledInput=DiscIntNeverNeededParam
  Gain : Gain  Gain=PLL_Ki
  Gain1 : Gain  Gain=PLL_Kd
  Gain2 : Gain  Gain=30/(pi*Pn)
  Mod : Math  Operator=mod
  Scope5 : Scope
  theta_pre : Outport
  speed_pre : Outport  Port=2
  wires:
  Discrete-Time Integrator/1 -> Add/1
  Gain1/1 -> Add/2
  Gain/1 -> Discrete-Time Integrator/1
  Gain2/1 -> speed_pre/1
  Constant2/1 -> Mod/2
  Discrete-Time Integrator1/1 -> Mod/1, Scope5/1
  Mod/1 -> theta_pre/1
  Analog Filter Design1/1 -> Data Type Conversion2/1
  Data Type Conversion1/1 -> Analog Filter Design1/1
  Data Type Conversion2/1 -> Gain2/1
  Add/1 -> Data Type Conversion1/1, Discrete-Time Integrator1/1
  e_l/1 -> Gain1/1, Gain/1

== system Square_HFI/FOC_Mode/HFI_Mode/SVPWM ==
  U_alpha : Inport
  U_beta : Inport  Port=2
  T_pwm : Inport  Port=3
  u_dc : Inport  Port=4
  Constant : Constant
  Duty_Caculator : Subsystem
  Gain : Gain  Gain=2
  Mux : Mux  Inputs=3
  Sector_Select : Subsystem
  Sum : Sum  Inputs=|-+
  T4_T6_Caculator : Subsystem
  X_Y_Z_Caculator : Subsystem
  Duty : Outport
  wires:
  U_alpha/1 -> X_Y_Z_Caculator/1(u_alpha), Sector_Select/1(u_alpha)
  U_beta/1 -> X_Y_Z_Caculator/2(u_beta), Sector_Select/2(u_beta)
  T_pwm/1 -> Duty_Caculator/4(T_pwm), T4_T6_Caculator/5(T_pwm), X_Y_Z_Caculator/3(T_pwm)
  u_dc/1 -> X_Y_Z_Caculator/4(U_dc)
  X_Y_Z_Caculator/1(X) -> T4_T6_Caculator/2(X)
  X_Y_Z_Caculator/2(Y) -> T4_T6_Caculator/3(Y)
  X_Y_Z_Caculator/3(Z) -> T4_T6_Caculator/4(Z)
  Sector_Select/1(N) -> T4_T6_Caculator/1(N), Duty_Caculator/1(N)
  T4_T6_Caculator/2(T6) -> Duty_Caculator/3(T6)
  T4_T6_Caculator/1(T4) -> Duty_Caculator/2(T4)
  Duty_Caculator/2(Dutyb) -> Mux/2
  Duty_Caculator/1(Dutya) -> Mux/1
  Duty_Caculator/3(Dutyc) -> Mux/3
  Sum/1 -> Duty/1
  Constant/1 -> Sum/2
  Mux/1 -> Gain/1
  Gain/1 -> Sum/1

== system Square_HFI/FOC_Mode/HFI_Mode/Speed_PI_Controller ==
  SpeedRef : Inport
  SpeedFd : Inport  Port=2
  PID Controller3 : slpidlib/PID Controller  Controller=PI  Form=Parallel  TimeDomain=Discrete-time  UseExternalTs=off  SampleTime=-1  IntegratorMethod=Forward Euler  FilterMethod=Forward Euler  ControllerParametersSource=internal  P=spd_kp  I=spd_ki  UseKiTs=off  D=0  N=100  UseFilter=on  TunerSelectOption=Transfer Function Based (PID Tuner App)  InitialConditionSource=internal  InitialConditionForIntegrator=0  InitialConditionForFilter=0  DifferentiatorICPrevScaledInput=0  ExternalReset=none  TrackingMode=off  Kt=1  LimitOutput=on  SatLimitsSource=internal  UpperSaturationLimit=3  LowerSaturationLimit=-3  LinearizeAsGain=on  AntiWindupMode=clamping  Kb=0.013  LimitIntegrator=off  UpperIntegratorSaturationLimit=inf  LowerIntegratorSaturationLimit=-inf  PGainOutDataTypeStr=single  PProdOutDataTypeStr=single  POutMin=[]  POutMax=[]  IGainOutDataTypeStr=single  IProdOutDataTypeStr=single  IOutMin=[]  IOutMax=[]  DOutMin=[]  DOutMax=[]  NOutMin=[]  NOutMax=[]  SumOutDataTypeStr=single  SumOutMin=[]  SumOutMax=[]  SaturationOutDataTypeStr=single  SaturationOutMin=[]  SaturationOutMax=[]  PParamMin=[]  PParamMax=[]  IParamMin=[]  IParamMax=[]  DParamMin=[]  DParamMax=[]  NParamMin=[]  NParamMax=[]  KbParamMin=[]  KbParamMax=[]  KtParamMin=[]  KtParamMax=[]  KbOutMin=[]  KbOutMax=[]  KtOutMin=[]  KtOutMax=[]  IntegratorOutMin=[]  IntegratorOutMax=[]  FilterOutMin=[]  FilterOutMax=[]  SumI1OutMin=[]  SumI1OutMax=[]  SumI2OutMin=[]  SumI2OutMax=[]  SumI3OutMin=[]  SumI3OutMax=[]  SumI4OutMin=[]  SumI4OutMax=[]  SumDOutMin=[]  SumDOutMax=[]  DifferentiatorOutMin=[]  DifferentiatorOutMax=[]  FilterDiffOutCoefMin=[]  FilterDiffOutCoefMax=[]  ReciprocalOutMin=[]  ReciprocalOutMax=[]  SumDenOutMin=[]  SumDenOutMax=[]  SumNumOutMin=[]  SumNumOutMax=[]  DivideOutMin=[]  DivideOutMax=[]  UdiffTsProdOutMin=[]  UdiffTsProdOutMax=[]  NTsProdOutMin=[]  NTsProdOutMax=[]  UintegralTsProdOutMin=[]  UintegralTsProdOutMax=[]  UngainTsProdOutMin=[]  UngainTsProdOutMax=[]  ClampingZeroOutDataTypeStr=Inherit: Inherit via back propagation  ClampingZeroOutMin=[]  ClampingZeroOutMax=[]  FilterDenConstantOutDataTypeStr=Inherit: Inherit via back propagation  FilterDenConstantOutMin=[]  FilterDenConstantOutMax=[]  PCopyOutDataTypeStr=Inherit: Inherit via back propagation  PCopyOutMin=[]  PCopyOutMax=[]  NCopyOutDataTypeStr=Inherit: Inherit via back propagation  NCopyOutMin=[]  NCopyOutMax=[]  IntegratorContinuousStateAttributes=''  IntegratorStateMustResolveToSignalObject=off  IntegratorRTWStateStorageClass=Auto  FilterContinuousStateAttributes=''  FilterStateMustResolveToSignalObject=off  FilterRTWStateStorageClass=Auto  ParallelPVariant=InternalParameters  IdealPVariant=Disabled  IVariant=InternalParameters  DVariant=Disabled  IntegratorVariant=Discrete  SatVariant=Enabled  AWVariant=DiscClampingParallel  PCopyVariant=Disabled  TRVariant=Disabled  FdbkBlocksVariant=Forward  IdealPFdbkVariant=Disabled  SatFdbkVariant=Disabled  DerivativeFilterVariant=Disabled  NVariant=Disabled  NCopyVariant=Disabled_SignalSpec  FilterICVariant=Disabled  IntegratorICVariant=InternalICs  ExternalResetVariant=Disabled  TRSumVariant=Passthrough  SumFdbkVariant=Disabled  SumVariant=Sum_PI  TsampFilterVariant=InternalTs  TsampNgainVariant=Passthrough  TsampIntegralVariant=Passthrough  ExternalSaturationOutDataTypeStr=single
  Sum2 : Sum  Inputs=|+-  AccumDataTypeStr=single  OutDataTypeStr=single
  iqRef : Outport
  wires:
  PID Controller3/1 -> iqRef/1
  SpeedRef/1 -> Sum2/1
  SpeedFd/1 -> Sum2/2
  Sum2/1 -> PID Controller3/1

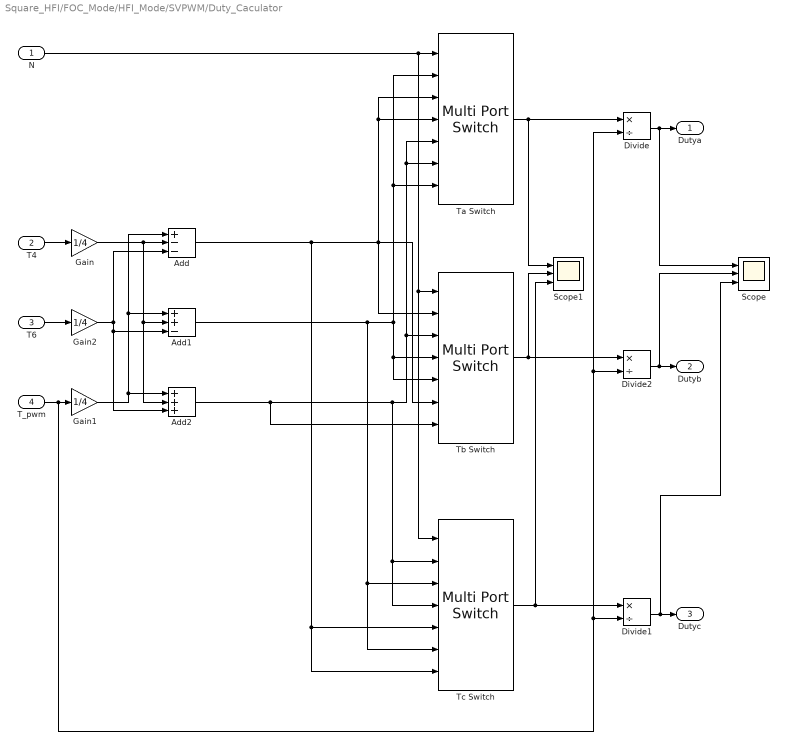
== system Square_HFI/FOC_Mode/HFI_Mode/SVPWM/Duty_Caculator ==
  N : Inport
  T4 : Inport  Port=2
  T6 : Inport  Port=3
  T_pwm : Inport  Port=4
  Add : Sum  Inputs=+--
  Add1 : Sum  Inputs=++-
  Add2 : Sum  Inputs=+++
  Divide : Product  Inputs=*/
  Divide1 : Product  Inputs=*/
  Divide2 : Product  Inputs=*/
  Gain : Gain  Gain=1/4
  Gain1 : Gain  Gain=1/4
  Gain2 : Gain  Gain=1/4
  Scope : Scope  NumInputPorts=3
  Scope1 : Scope  NumInputPorts=3
  Ta Switch : MultiPortSwitch  Inputs=6  DiagnosticForDefault=None  SaturateOnIntegerOverflow=off  InputSameDT=off
  Tb Switch : MultiPortSwitch  Inputs=6  DiagnosticForDefault=None  SaturateOnIntegerOverflow=off  InputSameDT=off
  Tc Switch : MultiPortSwitch  Inputs=6  DiagnosticForDefault=None  SaturateOnIntegerOverflow=off  InputSameDT=off
  Dutya : Outport
  Dutyb : Outport  Port=2
  Dutyc : Outport  Port=3
  wires:
  T4/1 -> Gain/1
  T6/1 -> Gain2/1
  T_pwm/1 -> Divide2/2, Divide/2, Divide1/2, Gain1/1
  Gain1/1 -> Add2/1, Add1/1, Add/1
  Gain/1 -> Add2/2, Add1/2, Add/2
  Gain2/1 -> Add2/3, Add1/3, Add/3
  N/1 -> Tc Switch/1, Tb Switch/1, Ta Switch/1
  Add/1 -> Tc Switch/7, Tc Switch/5, Tb Switch/6, Ta Switch/3, Ta Switch/4, Tb Switch/2
  Add1/1 -> Tc Switch/3, Tc Switch/6, Ta Switch/7, Ta Switch/2, Tb Switch/5, Tb Switch/4
  Add2/1 -> Tb Switch/7, Ta Switch/5, Ta Switch/6, Tb Switch/3, Tc Switch/4, Tc Switch/2
  Ta Switch/1 -> Scope1/1, Divide/1
  Tb Switch/1 -> Scope1/2, Divide2/1
  Tc Switch/1 -> Scope1/3, Divide1/1
  Divide/1 -> Scope/1, Dutya/1
  Divide1/1 -> Scope/3, Dutyc/1
  Divide2/1 -> Scope/2, Dutyb/1

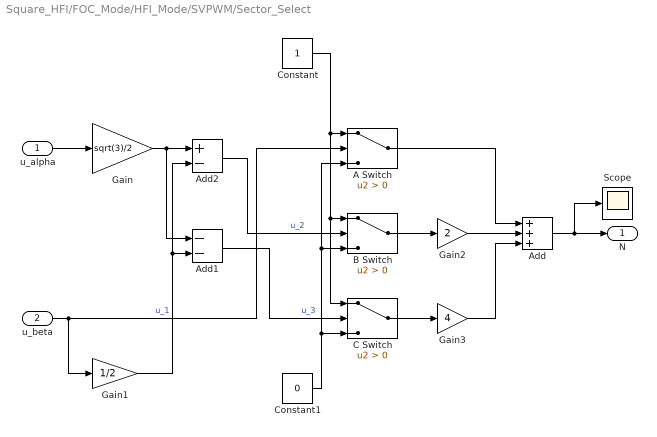
== system Square_HFI/FOC_Mode/HFI_Mode/SVPWM/Sector_Select ==
  u_alpha : Inport
  u_beta : Inport  Port=2
  " A Switch" : Switch  Criteria=u2 > Threshold  SaturateOnIntegerOverflow=off  InputSameDT=off
  " B Switch" : Switch  Criteria=u2 > Threshold  SaturateOnIntegerOverflow=off  InputSameDT=off
  " C Switch" : Switch  Criteria=u2 > Threshold  SaturateOnIntegerOverflow=off  InputSameDT=off
  Add : Sum  Inputs=+++
  Add1 : Sum  Inputs=--
  Add2 : Sum  Inputs=+-
  Constant : Constant
  Constant1 : Constant  Value=0
  Gain : Gain  Gain=sqrt(3)/2
  Gain1 : Gain  Gain=1/2
  Gain2 : Gain  Gain=2
  Gain3 : Gain  Gain=4
  Scope : Scope
  N : Outport
  wires:
  Constant/1 -> " C Switch"/1, " B Switch"/1, " A Switch"/1
  Constant1/1 -> " C Switch"/3, " B Switch"/3, " A Switch"/3
  " A Switch"/1 -> Add/1
  Add/1 -> Scope/1, N/1
  " C Switch"/1 -> Gain3/1
  " B Switch"/1 -> Gain2/1
  u_beta/1 -> Gain1/1, " A Switch"/2  "u_1"
  u_alpha/1 -> Gain/1
  Gain/1 -> Add1/1, Add2/1
  Gain1/1 -> Add1/2, Add2/2
  Add2/1 -> " B Switch"/2  "u_2"
  Add1/1 -> " C Switch"/2  "u_3"
  Gain2/1 -> Add/2
  Gain3/1 -> Add/3

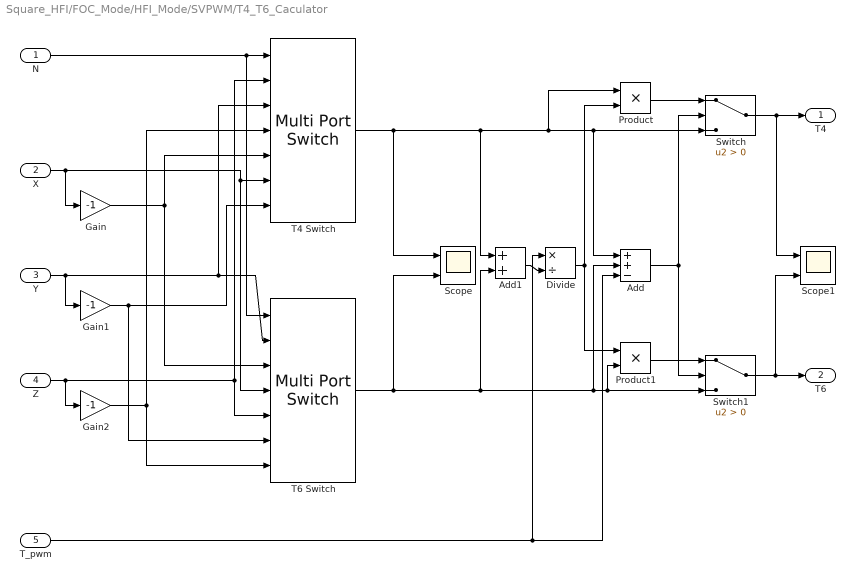
== system Square_HFI/FOC_Mode/HFI_Mode/SVPWM/T4_T6_Caculator ==
  N : Inport
  X : Inport  Port=2
  Y : Inport  Port=3
  Z : Inport  Port=4
  T_pwm : Inport  Port=5
  Add : Sum  Inputs=++-
  Add1 : Sum
  Divide : Product  Inputs=*/
  Gain : Gain  Gain=-1
  Gain1 : Gain  Gain=-1
  Gain2 : Gain  Gain=-1
  Product : Product
  Product1 : Product
  Scope : Scope  NumInputPorts=2
  Scope1 : Scope  NumInputPorts=2
  Switch : Switch  Criteria=u2 > Threshold  SaturateOnIntegerOverflow=off  InputSameDT=off
  Switch1 : Switch  Criteria=u2 > Threshold  SaturateOnIntegerOverflow=off  InputSameDT=off
  T4 Switch : MultiPortSwitch  Inputs=6  DiagnosticForDefault=None  SaturateOnIntegerOverflow=off  InputSameDT=off
  T6 Switch : MultiPortSwitch  Inputs=6  DiagnosticForDefault=None  SaturateOnIntegerOverflow=off  InputSameDT=off
  T4 : Outport
  T6 : Outport  Port=2
  wires:
  Z/1 -> T4 Switch/2, T6 Switch/5, Gain2/1
  Y/1 -> Gain1/1, T4 Switch/3, T6 Switch/2
  X/1 -> T4 Switch/6, T6 Switch/4, Gain/1
  N/1 -> T6 Switch/1, T4 Switch/1
  Gain/1 -> T6 Switch/3, T4 Switch/5
  Gain2/1 -> T6 Switch/7, T4 Switch/4
  Gain1/1 -> T4 Switch/7, T6 Switch/6
  T4 Switch/1 -> Add1/1, Product/1, Add/1, Switch/3, Scope/1
  T6 Switch/1 -> Add1/2, Add/2, Switch1/3, Product1/2, Scope/2
  T_pwm/1 -> Add/3, Divide/1
  Add/1 -> Switch1/2, Switch/2
  Add1/1 -> Divide/2
  Product1/1 -> Switch1/1
  Product/1 -> Switch/1
  Divide/1 -> Product/2, Product1/1
  Switch/1 -> Scope1/1, T4/1
  Switch1/1 -> Scope1/2, T6/1

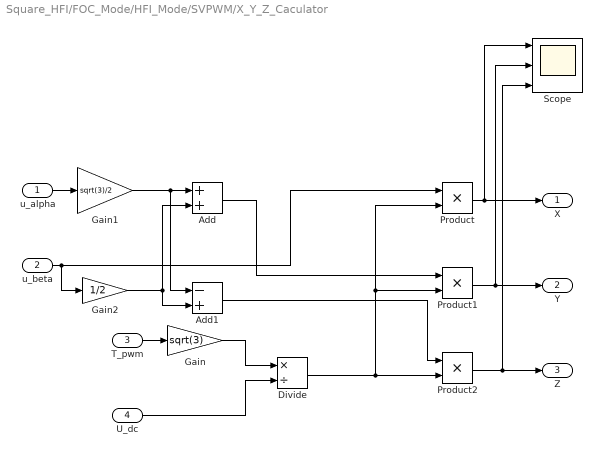
== system Square_HFI/FOC_Mode/HFI_Mode/SVPWM/X_Y_Z_Caculator ==
  u_alpha : Inport
  u_beta : Inport  Port=2
  T_pwm : Inport  Port=3
  U_dc : Inport  Port=4
  Add : Sum
  Add1 : Sum  Inputs=-+
  Divide : Product  Inputs=*/
  Gain : Gain  Gain=sqrt(3)
  Gain1 : Gain  Gain=sqrt(3)/2
  Gain2 : Gain  Gain=1/2
  Product : Product
  Product1 : Product
  Product2 : Product
  Scope : Scope  NumInputPorts=3
  X : Outport
  Y : Outport  Port=2
  Z : Outport  Port=3
  wires:
  T_pwm/1 -> Gain/1
  U_dc/1 -> Divide/2
  Gain/1 -> Divide/1
  u_beta/1 -> Gain2/1, Product/1
  Divide/1 -> Product2/2, Product1/2, Product/2
  Product/1 -> Scope/1, X/1
  u_alpha/1 -> Gain1/1
  Gain1/1 -> Add1/1, Add/1
  Gain2/1 -> Add1/2, Add/2
  Add/1 -> Product1/1
  Product1/1 -> Scope/2, Y/1
  Add1/1 -> Product2/1
  Product2/1 -> Scope/3, Z/1
